simulink model "test_quadruped_staticwalk"  (R2018b)
settings: Solver=ode4  StartTime=0.0  StopTime=5  FixedStep=0.001  RelTol=1e-3  EnableMultiTasking=on
values from neighbouring files (symbols this model uses):
  Matlab_version = str2double(r_temp___(1))    [quadruped.m]
  Output_File = 'quadruped_demo1'    [quadruped.m]
  Output_file_n = r_temp___(2)    [quadruped.m]
  Plant_inputs_num = r_temp___(1)    [quadruped.m]
  Plant_outputs_num = r_temp___(1)    [quadruped.m]
  RecurDyn = 'C:\Program Files\FunctionBay, Inc\RecurDyn V9R1\Bin\'    [quadruped.m]
  RecurDyn_controltimestep = 1.e-003    (= 0.001)    [quadruped.m]
  RecurDyn_model = 'quadruped_demo1'    [quadruped.m]
  RecurDyn_model_n = r_temp___(2)    [quadruped.m]
settings Model: Creator=Administrator  LastModifiedBy=ahl19
settings OptimizationCC: LifeSpan=inf
settings DebuggingCC: SFUnexpectedBacktrackingDiag=warning  SFNoUnconditionalDefaultTransitionDiag=warning
settings SFSimCC: SimUseLocalCustomCode=off
settings RTWCC: RTWUseLocalCustomCode=off
settings CodeAppCC: StateflowObjectComments=on
settings GRTTargetCC: TargetLangStandard=C89/C90 (ANSI)  GeneratePreprocessorConditionals=Disable all
settings ConfigComp: CovMetricSettings=dw  CovHtmlReporting=on  CovSaveCumulativeToWorkspaceVar=on  CovSaveSingleToWorkspaceVar=on  CovExternalEMLEnable=off

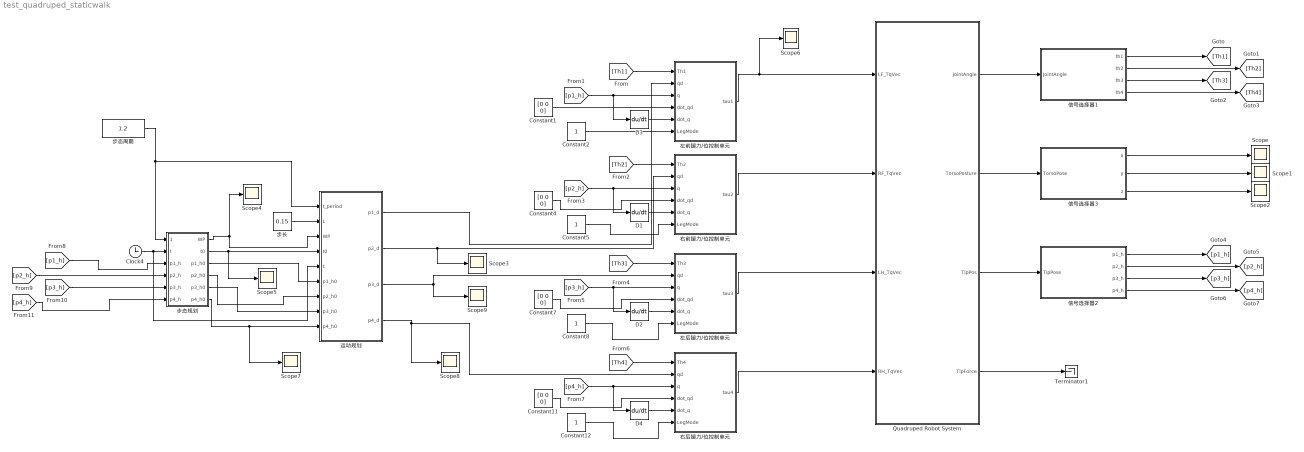
== system test_quadruped_staticwalk ==
  Clock4 : Clock
  Constant{1,4,7,11} (4 alike) : Constant  Value=[0 0 0]
  Constant{2,5,8,12} (4 alike) : Constant
  D{1..4} (4 alike) : Derivative  CoefficientInTFapproximation=0.01
  Quadruped Robot System : Subsystem
  Scope{,1..9} (10 alike) : Scope
  Terminator1 : Terminator
  信号选择器1 : MATLAB Function  TreatAsAtomicUnit=on
  信号选择器2 : MATLAB Function  TreatAsAtomicUnit=on
  信号选择器3 : MATLAB Function  TreatAsAtomicUnit=on
  右前腿力/位控制单元 : MATLAB Function  TreatAsAtomicUnit=on
  右后腿力/位控制单元 : MATLAB Function  TreatAsAtomicUnit=on
  左前腿力/位控制单元 : MATLAB Function  TreatAsAtomicUnit=on
  左后腿力/位控制单元 : MATLAB Function  TreatAsAtomicUnit=on
  步态周期 : Constant  Value=1.2
  步态规划 : MATLAB Function  TreatAsAtomicUnit=on
  步长 : Constant  Value=0.15
  运动规划 : MATLAB Function  TreatAsAtomicUnit=on
  wires:
  Quadruped Robot System/1(JointAngle) -> 信号选择器1/1(JointAngle)
  Quadruped Robot System/3(TipPos) -> 信号选择器2/1(TipPose)
  左前腿力/位控制单元/1(tau1) -> Scope6/1, Quadruped Robot System/1(LF_TqVec)
  右前腿力/位控制单元/1(tau2) -> Quadruped Robot System/2(RF_TqVec)
  左后腿力/位控制单元/1(tau3) -> Quadruped Robot System/3(LH_TqVec)
  右后腿力/位控制单元/1(tau4) -> Quadruped Robot System/4(RH_TqVec)
  信号选择器1/1(th1) -> [Th1]
  信号选择器1/2(th2) -> [Th2]
  信号选择器1/3(th3) -> [Th3]
  信号选择器1/4(th4) -> [Th4]
  [Th1] -> 左前腿力/位控制单元/1(Th1)
  信号选择器2/1(p1_h) -> [p1_h]
  信号选择器2/2(p2_h) -> [p2_h]
  信号选择器2/3(p3_h) -> [p3_h]
  信号选择器2/4(p4_h) -> [p4_h]
  [p1_h] -> D3/1, 左前腿力/位控制单元/3(q)
  Constant1/1 -> 左前腿力/位控制单元/4(dot_qd)
  D3/1 -> 左前腿力/位控制单元/5(dot_q)
  Constant2/1 -> 左前腿力/位控制单元/6(LegMode)
  [Th2] -> 右前腿力/位控制单元/1(Th2)
  [p2_h] -> 右前腿力/位控制单元/3(q), D1/1
  Constant4/1 -> 右前腿力/位控制单元/4(dot_qd)
  Constant5/1 -> 右前腿力/位控制单元/6(LegMode)
  [Th3] -> 左后腿力/位控制单元/1(Th3)
  [p3_h] -> 左后腿力/位控制单元/3(q), D2/1
  Constant7/1 -> 左后腿力/位控制单元/4(dot_qd)
  Constant8/1 -> 左后腿力/位控制单元/6(LegMode)
  D1/1 -> 右前腿力/位控制单元/5(dot_q)
  D2/1 -> 左后腿力/位控制单元/5(dot_q)
  [Th4] -> 右后腿力/位控制单元/1(Th4)
  [p4_h] -> 右后腿力/位控制单元/3(q), D4/1
  Constant11/1 -> 右后腿力/位控制单元/4(dot_qd)
  Constant12/1 -> 右后腿力/位控制单元/6(LegMode)
  D4/1 -> 右后腿力/位控制单元/5(dot_q)
  Quadruped Robot System/4(TipForce) -> Terminator1/1
  Quadruped Robot System/2(TorsoPosture) -> 信号选择器3/1(TorsoPose)
  信号选择器3/1(x) -> Scope/1
  信号选择器3/2(y) -> Scope1/1
  信号选择器3/3(z) -> Scope2/1
  Clock4/1 -> 步态规划/2(t), 运动规划/5(t)
  步态规划/1(WP) -> 运动规划/3(WP), Scope4/1
  步态规划/2(t0) -> Scope5/1, 运动规划/4(t0)
  步态周期/1 -> 运动规划/1(t_period), 步态规划/1(period)
  步长/1 -> 运动规划/2(L)
  [p1_h] -> 步态规划/3(p1_h)
  [p2_h] -> 步态规划/4(p2_h)
  [p3_h] -> 步态规划/5(p3_h)
  [p4_h] -> 步态规划/6(p4_h)
  步态规划/3(p1_h0) -> 运动规划/6(p1_h0)
  步态规划/4(p2_h0) -> 运动规划/7(p2_h0)
  步态规划/5(p3_h0) -> 运动规划/8(p3_h0)
  步态规划/6(p4_h0) -> Scope7/1, 运动规划/9(p4_h0)
  运动规划/1(p1_d) -> 左前腿力/位控制单元/2(qd)
  运动规划/2(p2_d) -> Scope3/1, 右前腿力/位控制单元/2(qd)
  运动规划/3(p3_d) -> Scope9/1, 左后腿力/位控制单元/2(qd)
  运动规划/4(p4_d) -> Scope8/1, 右后腿力/位控制单元/2(qd)

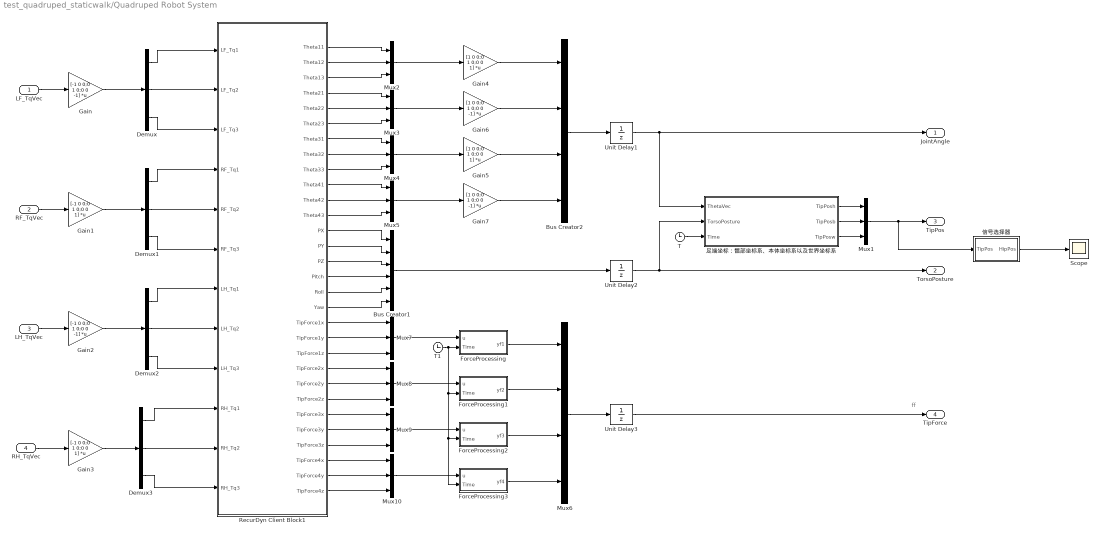
== system test_quadruped_staticwalk/Quadruped Robot System ==
  note: ff
  LF_TqVec : Inport
  RF_TqVec : Inport  Port=2
  LH_TqVec : Inport  Port=3
  RH_TqVec : Inport  Port=4
  Bus Creator1 : BusCreator  Inputs=6
  Bus Creator2 : BusCreator  Inputs=4
  Demux{,1..3} (4 alike) : Demux  Outputs=3
  ForceProcessing : MATLAB Function  TreatAsAtomicUnit=on
  ForceProcessing1 : MATLAB Function  TreatAsAtomicUnit=on
  ForceProcessing2 : MATLAB Function  TreatAsAtomicUnit=on
  ForceProcessing3 : MATLAB Function  TreatAsAtomicUnit=on
  Gain : Gain  Gain=[-1 0 0;0 1 0;0 0 -1]  Multiplication=Matrix(K*u) (u vector)
  Gain1 : Gain  Gain=[-1 0 0;0 1 0;0 0 1]  Multiplication=Matrix(K*u) (u vector)
  Gain2 : Gain  Gain=[-1 0 0;0 1 0;0 0 -1]  Multiplication=Matrix(K*u) (u vector)
  Gain3 : Gain  Gain=[-1 0 0;0 1 0;0 0 1]  Multiplication=Matrix(K*u) (u vector)
  Gain4 : Gain  Gain=[1 0 0;0 1 0;0 0 1]  Multiplication=Matrix(K*u) (u vector)
  Gain5 : Gain  Gain=[1 0 0;0 1 0;0 0 1]  Multiplication=Matrix(K*u) (u vector)
  Gain6 : Gain  Gain=[1 0 0;0 1 0;0 0 -1]  Multiplication=Matrix(K*u) (u vector)
  Gain7 : Gain  Gain=[1 0 0;0 1 0;0 0 -1]  Multiplication=Matrix(K*u) (u vector)
  Mux{1..5,7..10} (9 alike) : Mux  Inputs=3
  Mux6 : Mux
  RecurDyn Client Block1 : Subsystem
      mask Display: image(imread('RecurDyn_IF3x_Client.jpg'))
  Scope : Scope
  T : Clock
  T1 : Clock
  Unit Delay1 : UnitDelay  InitialCondition=[pi/2;pi/4;0;pi/2;pi/4;0;pi/2;pi/4;0;pi/2;pi/4;0]  SampleTime=0.001
  Unit Delay2 : UnitDelay  InitialCondition=[0;0.70;0;0;0;0]  SampleTime=0.001
  Unit Delay3 : UnitDelay  InitialCondition=[0;0;0;0;0;0;0;0;0;0;0;0]  SampleTime=0.001
  信号选择器 : MATLAB Function  TreatAsAtomicUnit=on
  足端坐标：髋部坐标系、本体坐标系以及世界坐标系 : MATLAB Function  TreatAsAtomicUnit=on
  JointAngle : Outport
  TorsoPosture : Outport  Port=2
  TipPos : Outport  Port=3
  TipForce : Outport  Port=4
  wires:
  Bus Creator2/1 -> Unit Delay1/1
  Mux1/1 -> 信号选择器/1(TipPos), TipPos/1
  足端坐标：髋部坐标系、本体坐标系以及世界坐标系/1(TipPosh) -> Mux1/1
  足端坐标：髋部坐标系、本体坐标系以及世界坐标系/2(TipPosb) -> Mux1/2
  足端坐标：髋部坐标系、本体坐标系以及世界坐标系/3(TipPosw) -> Mux1/3
  Unit Delay1/1 -> JointAngle/1, 足端坐标：髋部坐标系、本体坐标系以及世界坐标系/1(ThetaVec)
  Unit Delay3/1 -> TipForce/1
  Unit Delay2/1 -> TorsoPosture/1, 足端坐标：髋部坐标系、本体坐标系以及世界坐标系/2(TorsoPosture)
  Mux7/1 -> ForceProcessing/1(u)
  Mux8/1 -> ForceProcessing1/1(u)
  Mux9/1 -> ForceProcessing2/1(u)
  Mux10/1 -> ForceProcessing3/1(u)
  Gain/1 -> Demux/1
  LF_TqVec/1 -> Gain/1
  RF_TqVec/1 -> Gain1/1
  LH_TqVec/1 -> Gain2/1
  RH_TqVec/1 -> Gain3/1
  Mux2/1 -> Gain4/1
  Bus Creator1/1 -> Unit Delay2/1
  Demux/2 -> RecurDyn Client Block1/2(LF_Tq2)
  RecurDyn Client Block1/1("Theta11   ") -> Mux2/1
  RecurDyn Client Block1/2("Theta12   ") -> Mux2/2
  RecurDyn Client Block1/3("Theta13   ") -> Mux2/3
  RecurDyn Client Block1/4("Theta21   ") -> Mux3/1
  RecurDyn Client Block1/5("Theta22   ") -> Mux3/2
  RecurDyn Client Block1/6("Theta23   ") -> Mux3/3
  Mux3/1 -> Gain6/1
  RecurDyn Client Block1/7("Theta31   ") -> Mux4/1
  RecurDyn Client Block1/8("Theta32   ") -> Mux4/2
  RecurDyn Client Block1/9("Theta33   ") -> Mux4/3
  RecurDyn Client Block1/10("Theta41   ") -> Mux5/1
  RecurDyn Client Block1/11("Theta42   ") -> Mux5/2
  RecurDyn Client Block1/12("Theta43   ") -> Mux5/3
  Mux4/1 -> Gain5/1
  Mux5/1 -> Gain7/1
  Demux1/2 -> RecurDyn Client Block1/5(RF_Tq2)
  Demux1/1 -> RecurDyn Client Block1/4(RF_Tq1)
  Demux1/3 -> RecurDyn Client Block1/6(RF_Tq3)
  Demux/1 -> RecurDyn Client Block1/1(LF_Tq1)
  Demux/3 -> RecurDyn Client Block1/3(LF_Tq3)
  Gain1/1 -> Demux1/1
  Demux2/2 -> RecurDyn Client Block1/8(LH_Tq2)
  Demux2/1 -> RecurDyn Client Block1/7(LH_Tq1)
  Demux2/3 -> RecurDyn Client Block1/9(LH_Tq3)
  Gain2/1 -> Demux2/1
  Demux3/2 -> RecurDyn Client Block1/11(RH_Tq2)
  Demux3/1 -> RecurDyn Client Block1/10(RH_Tq1)
  Demux3/3 -> RecurDyn Client Block1/12(RH_Tq3)
  Gain3/1 -> Demux3/1
  RecurDyn Client Block1/19(TipForce1x) -> Mux7/1
  RecurDyn Client Block1/20(TipForce1y) -> Mux7/2
  RecurDyn Client Block1/21(TipForce1z) -> Mux7/3
  RecurDyn Client Block1/22(TipForce2x) -> Mux8/1
  RecurDyn Client Block1/23(TipForce2y) -> Mux8/2
  RecurDyn Client Block1/24(TipForce2z) -> Mux8/3
  RecurDyn Client Block1/25(TipForce3x) -> Mux9/1
  RecurDyn Client Block1/26(TipForce3y) -> Mux9/2
  RecurDyn Client Block1/27(TipForce3z) -> Mux9/3
  RecurDyn Client Block1/28(TipForce4x) -> Mux10/1
  RecurDyn Client Block1/29(TipForce4y) -> Mux10/2
  RecurDyn Client Block1/30(TipForce4z) -> Mux10/3
  RecurDyn Client Block1/13("PX        ") -> Bus Creator1/1
  RecurDyn Client Block1/14("PY        ") -> Bus Creator1/2
  RecurDyn Client Block1/15("PZ        ") -> Bus Creator1/3
  RecurDyn Client Block1/16("Pitch     ") -> Bus Creator1/4
  RecurDyn Client Block1/17("Roll      ") -> Bus Creator1/5
  RecurDyn Client Block1/18("Yaw       ") -> Bus Creator1/6
  Gain4/1 -> Bus Creator2/1
  Gain6/1 -> Bus Creator2/2
  Gain5/1 -> Bus Creator2/3
  Gain7/1 -> Bus Creator2/4
  Mux6/1 -> Unit Delay3/1
  T/1 -> 足端坐标：髋部坐标系、本体坐标系以及世界坐标系/3(Time)
  ForceProcessing/1(yf1) -> Mux6/1
  ForceProcessing1/1(yf2) -> Mux6/2
  ForceProcessing2/1(yf3) -> Mux6/3
  ForceProcessing3/1(yf4) -> Mux6/4
  T1/1 -> ForceProcessing/2(Time), ForceProcessing1/2(Time), ForceProcessing2/2(Time), ForceProcessing3/2(Time)
  信号选择器/1(HipPos) -> Scope/1

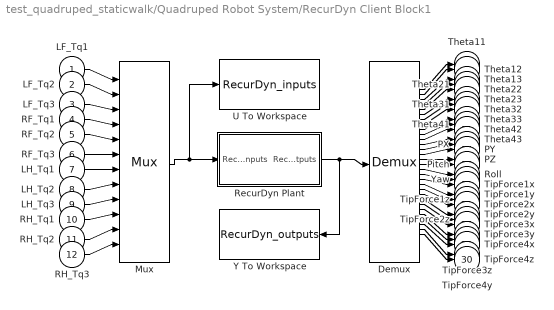
== system test_quadruped_staticwalk/Quadruped Robot System/RecurDyn Client Block1 ==
  LF_Tq1 : Inport
  LF_Tq2 : Inport  Port=2
  LF_Tq3 : Inport  Port=3
  RF_Tq1 : Inport  Port=4
  RF_Tq2 : Inport  Port=5
  RF_Tq3 : Inport  Port=6
  LH_Tq1 : Inport  Port=7
  LH_Tq2 : Inport  Port=8
  LH_Tq3 : Inport  Port=9
  RH_Tq1 : Inport  Port=10
  RH_Tq2 : Inport  Port=11
  RH_Tq3 : Inport  Port=12
  Demux : Demux  Outputs=30
  Mux : Mux  Inputs=12
  RecurDyn Plant : Subsystem  mask(Recurdyn/Plant){RecurDyn_model_name=RecurDyn_model, Output_File_Name_=Output_File, RecurDyn_=RecurDyn, Matlab_version_=Matlab_version, RecurDyn_controltimestep_=RecurDyn_controltimestep, RecurDyn_step_=100, Waitingtime=1000, RecurDyn_static_=off, RecurDyn_show_=on, RecurDyn_ani_=on, Create_Output_Folder_=off}
      mask prompts: Output_File_Name_ "Output File Name"; RecurDyn_ "RecurDyn_install_directory"; Matlab_version_ "Matlab version"; RecurDyn_controltimestep_ "Sampling period"; RecurDyn_step_ "RecurDyn_step"; Waitingtime "Waiting time"; RecurDyn_static_ "Static analysis"; RecurDyn_show_ "RecurDyn_show"; RecurDyn_ani_ "RecurDyn_animation"; Create_Output_Folder_ "Create Output Folder"
      mask help:
      | Simulate any Recurdyn Dynamics Model in Recurdyn/Solver
      | Plant inputs and Plant outputs are transfered every sampling time
      | Here, sampling time is determined by sampling period (Control time step)
      mask Display: disp( 'Dynamic Model' )
  U To Workspace : ToWorkspace  VariableName=RecurDyn_inputs
  Y To Workspace : ToWorkspace  VariableName=RecurDyn_outputs
  "Theta11   " : Outport
  "Theta12   " : Outport  Port=2
  "Theta13   " : Outport  Port=3
  "Theta21   " : Outport  Port=4
  "Theta22   " : Outport  Port=5
  "Theta23   " : Outport  Port=6
  "Theta31   " : Outport  Port=7
  "Theta32   " : Outport  Port=8
  "Theta33   " : Outport  Port=9
  "Theta41   " : Outport  Port=10
  "Theta42   " : Outport  Port=11
  "Theta43   " : Outport  Port=12
  "PX        " : Outport  Port=13
  "PY        " : Outport  Port=14
  "PZ        " : Outport  Port=15
  "Pitch     " : Outport  Port=16
  "Roll      " : Outport  Port=17
  "Yaw       " : Outport  Port=18
  TipForce1x : Outport  Port=19
  TipForce1y : Outport  Port=20
  TipForce1z : Outport  Port=21
  TipForce2x : Outport  Port=22
  TipForce2y : Outport  Port=23
  TipForce2z : Outport  Port=24
  TipForce3x : Outport  Port=25
  TipForce3y : Outport  Port=26
  TipForce3z : Outport  Port=27
  TipForce4x : Outport  Port=28
  TipForce4y : Outport  Port=29
  TipForce4z : Outport  Port=30
  wires:
  RecurDyn Plant/1(RecurDyn_outputs) -> Demux/1, Y To Workspace/1
  Mux/1 -> RecurDyn Plant/1(" RecurDyn_inputs"), U To Workspace/1
  Demux/1 -> "Theta11   "/1
  Demux/2 -> "Theta12   "/1
  Demux/3 -> "Theta13   "/1
  Demux/4 -> "Theta21   "/1
  Demux/5 -> "Theta22   "/1
  Demux/6 -> "Theta23   "/1
  Demux/7 -> "Theta31   "/1
  Demux/8 -> "Theta32   "/1
  Demux/9 -> "Theta33   "/1
  Demux/10 -> "Theta41   "/1
  Demux/11 -> "Theta42   "/1
  Demux/12 -> "Theta43   "/1
  Demux/13 -> "PX        "/1
  Demux/14 -> "PY        "/1
  Demux/15 -> "PZ        "/1
  Demux/16 -> "Pitch     "/1
  Demux/17 -> "Roll      "/1
  Demux/18 -> "Yaw       "/1
  Demux/19 -> TipForce1x/1
  Demux/20 -> TipForce1y/1
  Demux/21 -> TipForce1z/1
  Demux/22 -> TipForce2x/1
  Demux/23 -> TipForce2y/1
  Demux/24 -> TipForce2z/1
  Demux/25 -> TipForce3x/1
  Demux/26 -> TipForce3y/1
  Demux/27 -> TipForce3z/1
  Demux/28 -> TipForce4x/1
  Demux/29 -> TipForce4y/1
  Demux/30 -> TipForce4z/1
  LF_Tq1/1 -> Mux/1
  LF_Tq2/1 -> Mux/2
  LF_Tq3/1 -> Mux/3
  RF_Tq1/1 -> Mux/4
  RF_Tq2/1 -> Mux/5
  RF_Tq3/1 -> Mux/6
  LH_Tq1/1 -> Mux/7
  LH_Tq2/1 -> Mux/8
  LH_Tq3/1 -> Mux/9
  RH_Tq1/1 -> Mux/10
  RH_Tq2/1 -> Mux/11
  RH_Tq3/1 -> Mux/12

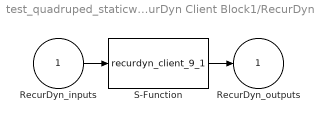
== system test_quadruped_staticwalk/Quadruped Robot System/RecurDyn Client Block1/RecurDyn Plant ==
  " RecurDyn_inputs" : Inport
  S-Function : S-Function  FunctionName=recurdyn_client_9_1  Parameters=RecurDyn_controltimestep_,RecurDyn_model_name,RecurDyn_,RecurDyn_static_,RecurDyn_step_,RecurDyn_show_,RecurDyn_ani_,Matlab_version_,RecurDyn_model_n,Plant_inputs_num,Plant_outputs_num,Waitingtime,Create_Output_Folder_,Output_File_Name_,Output_file_n  SFunctionDeploymentMode=off  EnableBusSupport=off
  RecurDyn_outputs : Outport  InitialOutput=0
  wires:
  S-Function/1 -> RecurDyn_outputs/1
  " RecurDyn_inputs"/1 -> S-Function/1

== matlab function test_quadruped_staticwalk/Quadruped Robot System/ForceProcessing1 ==
  data: u input; yf2 output; Time input
function yf2 = fp(u, Time)
% 处理足端力，y方向只提供大等于零的力
if Time<=0.001
    yf2 = zeros(3,1);
else
    yf2 = [1 0 0;0 (u(2)>=0) 0;0 0 1]*u;
end

end

== matlab function test_quadruped_staticwalk/Quadruped Robot System/ForceProcessing ==
  data: u input; yf1 output; Time input
function yf1 = fp(u, Time)
% 处理足端力，y方向只提供大等于零的力
if Time<=0.001
    yf1 = zeros(3,1);
else
    yf1 = [1 0 0;0 (u(2)>=0) 0;0 0 1]*u;
end

end

== matlab function test_quadruped_staticwalk/Quadruped Robot System/ForceProcessing2 ==
  data: u input; yf3 output; Time input
function yf3 = fp(u, Time)
% 处理足端力，y方向只提供大等于零的力
if Time<=0.001
    yf3 = zeros(3,1);
else
    yf3 = [1 0 0;0 (u(2)>=0) 0;0 0 1]*u;
end

end

== matlab function test_quadruped_staticwalk/Quadruped Robot System/ForceProcessing3 ==
  data: u input; yf4 output; Time input
function yf4 = fp(u, Time)
% 处理足端力，y方向只提供大等于零的力
if Time<=0.001
    yf4 = zeros(3,1);
else
    yf4 = [1 0 0;0 (u(2)>=0) 0;0 0 1]*u;
end

end

== matlab function test_quadruped_staticwalk/信号选择器2 ==
  data: TipPose input; p1_h output; p2_h output; p3_h output; p4_h output
function [p1_h,p2_h,p3_h,p4_h]  = SS(TipPose)

%% 
p1_h = TipPose(1:3);
p2_h = TipPose(4:6);
p3_h = TipPose(7:9);
p4_h = TipPose(10:12);


end

== matlab function test_quadruped_staticwalk/Quadruped Robot System/足端坐标：髋部坐标系、本体坐标系以及世界坐标系 ==
  data: ThetaVec input; TipPosh output; TipPosb output; TorsoPosture input; TipPosw output; Time input
function [TipPosh,TipPosb, TipPosw] = fk(ThetaVec, TorsoPosture, Time)

%% Notes
% 惯性系或世界坐标系：以机器人前进方向为【+X】，竖直向上为【+Y】，【+Z】由右手法则确定
% 本体固连坐标系：原点在质心处或几何中心，初始方向与惯性系一致
% 在髋部安装点处建立固连坐标系（方向与本体固连坐标系一致），计算足端位置（以下的顺序均为：左前、右前、左后、右后）

% BY ZPP
% 20171122

%% 设置仿真初值
if Time<=0.001
    ThetaVec = [pi/2;pi/4;0; pi/2;pi/4;0; pi/2;pi/4;0; pi/2;pi/4;0];
    TorsoPosture = [0; 0.70; 0;0;0;0];
end

%% 设置模型参数

% 重力加速度
g = 9.80665;

%本体尺寸的一半
L = 0.425; W = 0.19; H = -0.10 ;
% 本体质量
Mb = 50;

% 髋部安装点在本体固连坐标系中的坐标
A1 = [L -H -W]';
A2 = [L -H W]';
A3 = [-L -H -W]';
A4 = [-L -H W]';

Ab= [A1;A2;A3;A4];

% 单腿各连杆长度和质量
L1 = 0.35*sqrt(2);      % M1 = 1.0;
L2 = 0.35*sqrt(2);      % M2 = 1.5;
R3 = 0.06;                  % M3 = 0.5;

%% 输入关节角度
th11 = ThetaVec(1);
th12 = ThetaVec(2);
th13 = ThetaVec(3);

th21 = ThetaVec(4);
th22 = ThetaVec(5);
th23 = ThetaVec(6);

th31 = ThetaVec(7);
th32 = ThetaVec(8);
th33 = ThetaVec(9);

th41 = ThetaVec(10);
th42 = ThetaVec(11);
th43 = ThetaVec(12);

%% 正运动学1：计算髋部固连坐标系下足端的位置
x1 = L1*cos(th11 - th12) - L2*cos(th12);
y1 = - cos(th13)*(L2*sin(th12) + L1*sin(th11 - th12));
z1 = - sin(th13)*(L2*sin(th12) + L1*sin(th11 - th12));

x2 = L1*cos(th21 - th22) - L2*cos(th22);
y2 = - cos(th23)*(L2*sin(th22) + L1*sin(th21 - th22));
z2 = sin(th23)*(L2*sin(th22) + L1*sin(th21 - th22));

x3 = L1*cos(th31 - th32) - L2*cos(th32);
y3 = - cos(th33)*(L2*sin(th32) + L1*sin(th31 - th32));
z3 = - sin(th33)*(L2*sin(th32) + L1*sin(th31 - th32));

x4 = L1*cos(th41 - th42) - L2*cos(th42);
y4 = - cos(th43)*(L2*sin(th42) + L1*sin(th41 - th42));
z4 = sin(th43)*(L2*sin(th42) + L1*sin(th41 - th42));

TipPosh = [x1 y1 z1 x2 y2 z2 x3 y3 z3 x4 y4 z4]';

%% 正运动学2：计算本体固连坐标系下足端的位置
TipPosb = TipPosh + Ab;

%% 正运动学3：计算原点在本体质心处的惯性系下足端的位置
% 本体姿态角：Y-pitch / X-roll / Z-yaw
alpha = TorsoPosture(6); beta = TorsoPosture(4); gama = TorsoPosture(5);
RR = [cos(alpha)*cos(beta)  cos(alpha)*sin(beta)*sin(gama)-sin(alpha)*cos(gama)  cos(alpha)*sin(beta)*cos(gama)+sin(alpha)*sin(gama);...
         sin(alpha)*cos(beta)  sin(alpha)*sin(beta)*sin(gama)+cos(alpha)*cos(gama)  sin(alpha)*sin(beta)*cos(gama)-cos(alpha)*sin(gama);...
         -sin(beta)  cos(beta)*sin(gama)  cos(beta)*cos(gama)];
Rmat = blkdiag(RR,RR,RR,RR);
TipPosw = Rmat*TipPosb;

end

== matlab function test_quadruped_staticwalk/信号选择器3 ==
  data: TorsoPose input; x output; y output; z output
function [x,y,z]  = SS(TorsoPose)

%% 
x = TorsoPose(1);
y = TorsoPose(2);
z = TorsoPose(3);


end

== matlab function test_quadruped_staticwalk/右前腿力//位控制单元 ==
  data: Th2 input; qd input; q input; dot_qd input; dot_q input; LegMode input; tau2 output
%function [tau2,Fr]  = SLC(Th2,qd,q,dot_qd,dot_q,LegMode, Fwd,Fwf)
function tau2   = SLC(Th2,qd,q,dot_qd,dot_q,LegMode)

%% 关节角度、足端广义坐标以及雅克比矩阵的计算
th21=Th2(1);
th22=Th2(2);
th23=Th2(3);

% 单腿连杆参数
L1 = 0.35*sqrt(2);
L2 = 0.35*sqrt(2);
R3 = 0.06;

% Jacobian Matrix
J2 = [ -L1*sin(th21 - th22),                   L2*sin(th22) + L1*sin(th21 - th22),                      0;...
          -L1*cos(th21 - th22)*cos(th23), -cos(th23)*(L2*cos(th22) - L1*cos(th21 - th22)), sin(th23)*(L2*sin(th22) + L1*sin(th21 - th22));...
          L1*cos(th21 - th22)*sin(th23),   sin(th23)*(L2*cos(th22) - L1*cos(th21 - th22)),    cos(th23)*(L2*sin(th22) + L1*sin(th21 - th22))];

%% 初始化
 %Fr=zeros(3,1);
 %Fe = Fwf(4:6);    % 左前腿的足端接触力
 %Fd = Fwd(4:6);
 
tau2=zeros(3,1);

%% 单腿力/位控制模式
y = LegMode;
switch(y)
%%%%%%%%%%%%%%%%%%%%%%%%%%%%%
    

%%%%%%%%%%%%%%%%%%%%%%%%%%%%%
    case 1    % 单腿摆动
        kp = diag([8000 8000 8000]);
        kd = diag([500 500 500]);
        
        Fr=zeros(3,1);
        tau2=J2'*(kp*(qd-q)+kd*(dot_qd-dot_q)); 
        
%%%%%%%%%%%%%%%%%%%%%%%%%%%%%
    case 0    % 落后着地
        kp = diag([1000 1500 1000]);
        kd = diag([20 30 20]);
        
        % 在y方向上补偿0.01m
        qd1= qd+[0;-0.01;0];     
        Fr=zeros(3,1);
        tau2=J2'*(kp*(qd1-q)+kd*(dot_qd-dot_q));

%%%%%%%%%%%%%%%%%%%%%%%%%%%%%
     
end

%% 考虑实际情况：输出力矩限幅
Tmax = 500;

if tau2(1)>=Tmax
    tau2(1)=Tmax;
end
if tau2(1)<=-Tmax
    tau2(1)=-Tmax;
end
    
if tau2(2)>=Tmax
    tau2(2)=Tmax;
end
if tau2(2)<=-Tmax
    tau2(2)=-Tmax;
end
    
if tau2(3)>=Tmax
    tau2(3)=Tmax;
end
if tau2(3)<=-Tmax
    tau2(3)=-Tmax;
end

end

== matlab function test_quadruped_staticwalk/左后腿力//位控制单元 ==
  data: Th3 input; qd input; q input; dot_qd input; dot_q input; LegMode input; tau3 output
%function [tau3,Fr]  = SLC(Th3,qd,q,dot_qd,dot_q,LegMode, Fwd,Fwf)
function tau3   = SLC(Th3,qd,q,dot_qd,dot_q,LegMode)

%% 关节角度、足端广义坐标以及雅克比矩阵的计算
th31=Th3(1);
th32=Th3(2);
th33=Th3(3);

% 单腿连杆参数
L1 = 0.35*sqrt(2);
L2 = 0.35*sqrt(2);
R3 = 0.06;

% Jacobian Matrix
J3 = [ -L1*sin(th31 - th32),                   L2*sin(th32) + L1*sin(th31 - th32),                      0;...
          -L1*cos(th31 - th32)*cos(th33), -cos(th33)*(L2*cos(th32) - L1*cos(th31 - th32)), sin(th33)*(L2*sin(th32) + L1*sin(th31 - th32));...
          -L1*cos(th31 - th32)*sin(th33),  -sin(th33)*(L2*cos(th32) - L1*cos(th31 - th32)),  - cos(th33)*(L2*sin(th32) + L1*sin(th31 - th32))];

%% 初始化
 %Fr=zeros(3,1);
 %Fe = Fwf(7:9);    % 左前腿的足端接触力
 %Fd = Fwd(7:9);
 
tau3=zeros(3,1);

%% 单腿力/位控制模式
y = LegMode;
switch(y)
%%%%%%%%%%%%%%%%%%%%%%%%%%%%%
   

%%%%%%%%%%%%%%%%%%%%%%%%%%%%%
    case 1    % 单腿摆动
        kp = diag([8000 8000 8000]);
        kd = diag([500 500 500]);
        
        Fr=zeros(3,1);
        tau3=J3'*(kp*(qd-q)+kd*(dot_qd-dot_q)); 
        
%%%%%%%%%%%%%%%%%%%%%%%%%%%%%
    case 0    % 落后着地
        kp = diag([1000 1500 1000]);
        kd = diag([20 30 20]);
        
        % 在y方向上补偿0.01m
        qd1= qd+[0;-0.01;0];     
        Fr=zeros(3,1);
        tau3=J3'*(kp*(qd1-q)+kd*(dot_qd-dot_q));

%%%%%%%%%%%%%%%%%%%%%%%%%%%%%
     
end

%% 考虑实际情况：输出力矩限幅
Tmax = 500;

if tau3(1)>=Tmax
    tau3(1)=Tmax;
end
if tau3(1)<=-Tmax
    tau3(1)=-Tmax;
end
    
if tau3(2)>=Tmax
    tau3(2)=Tmax;
end
if tau3(2)<=-Tmax
    tau3(2)=-Tmax;
end
    
if tau3(3)>=Tmax
    tau3(3)=Tmax;
end
if tau3(3)<=-Tmax
    tau3(3)=-Tmax;
end

end

== matlab function test_quadruped_staticwalk/右后腿力//位控制单元 ==
  data: Th4 input; qd input; q input; dot_qd input; dot_q input; LegMode input; tau4 output
%function [tau4,Fr]  = SLC(Th4,qd,q,dot_qd,dot_q,LegMode, Fwd,Fwf)
function tau4   = SLC(Th4,qd,q,dot_qd,dot_q,LegMode)

%% 关节角度、足端广义坐标以及雅克比矩阵的计算
th41=Th4(1);
th42=Th4(2);
th43=Th4(3);

% 单腿连杆参数
L1 = 0.35*sqrt(2);
L2 = 0.35*sqrt(2);
R3 = 0.06;

% Jacobian Matrix
J4 = [ -L1*sin(th41 - th42),                   L2*sin(th42) + L1*sin(th41 - th42),                      0;...
          -L1*cos(th41 - th42)*cos(th43), -cos(th43)*(L2*cos(th42) - L1*cos(th41 - th42)), sin(th43)*(L2*sin(th42) + L1*sin(th41 - th42));...
          L1*cos(th41 - th42)*sin(th43),   sin(th43)*(L2*cos(th42) - L1*cos(th41 - th42)),    cos(th43)*(L2*sin(th42) + L1*sin(th41 - th42))];

%% 初始化
% Fr=zeros(3,1);
% Fe = Fwf(10:12);    % 左前腿的足端接触力
% Fd = Fwd(10:12);
 
tau4=zeros(3,1);

%% 单腿力/位控制模式
y = LegMode;
switch(y)
%%%%%%%%%%%%%%%%%%%%%%%%%%%%%
    

%%%%%%%%%%%%%%%%%%%%%%%%%%%%%
    case 1    % 单腿摆动
        kp = diag([8000 8000 8000]);
        kd = diag([500 500 500]);
        
        Fr=zeros(3,1);
        tau4=J4'*(kp*(qd-q)+kd*(dot_qd-dot_q)); 
        
%%%%%%%%%%%%%%%%%%%%%%%%%%%%%
    case 0    % 落后着地
        kp = diag([1000 1500 1000]);
        kd = diag([20 30 20]);
        
        % 在y方向上补偿0.01m
        qd1= qd+[0;-0.01;0];     
        Fr=zeros(3,1);
        tau4=J4'*(kp*(qd1-q)+kd*(dot_qd-dot_q));

%%%%%%%%%%%%%%%%%%%%%%%%%%%%%
     
end

%% 考虑实际情况：输出力矩限幅
Tmax = 500;

if tau4(1)>=Tmax
    tau4(1)=Tmax;
end
if tau4(1)<=-Tmax
    tau4(1)=-Tmax;
end
    
if tau4(2)>=Tmax
    tau4(2)=Tmax;
end
if tau4(2)<=-Tmax
    tau4(2)=-Tmax;
end
    
if tau4(3)>=Tmax
    tau4(3)=Tmax;
end
if tau4(3)<=-Tmax
    tau4(3)=-Tmax;
end

end

== matlab function test_quadruped_staticwalk/Quadruped Robot System/信号选择器 ==
  data: TipPos input; HipPos output
function HipPos  = SS(TipPos)

%% 
HipPos = TipPos(1:3);


end

== matlab function test_quadruped_staticwalk/左前腿力//位控制单元 ==
  data: Th1 input; qd input; q input; dot_qd input; dot_q input; LegMode input; tau1 output
%function [tau1,Fr, Fe]  = SLC(Th1,qd,q,dot_qd,dot_q,LegMode, Fwd,Fwf)
function tau1   = SLC(Th1,qd,q,dot_qd,dot_q,LegMode)

%% 关节角度、足端广义坐标以及雅克比矩阵的计算
th11=Th1(1);
th12=Th1(2);
th13=Th1(3);

% 单腿连杆参数
L1 = 0.35*sqrt(2);
L2 = 0.35*sqrt(2);
R3 = 0.06;

% Jacobian Matrix
J1 = [ -L1*sin(th11 - th12),                   L2*sin(th12) + L1*sin(th11 - th12),                      0;...
          -L1*cos(th11 - th12)*cos(th13), -cos(th13)*(L2*cos(th12) - L1*cos(th11 - th12)), sin(th13)*(L2*sin(th12) + L1*sin(th11 - th12));...
          -L1*cos(th11 - th12)*sin(th13),  -sin(th13)*(L2*cos(th12) - L1*cos(th11 - th12)),  - cos(th13)*(L2*sin(th12) + L1*sin(th11 - th12))];

%% 初始化
 %Fr=zeros(3,1);
 %Fe = Fwf(1:3);    % 左前腿的足端接触力
 %Fd = Fwd(1:3);
 
tau1=zeros(3,1);


%% 单腿力/位控制模式
y = LegMode;            %LegMode：0为落后着地模式；1为单腿摆动模式；2为单腿支撑模式；3为提前着地模式
switch(y)
%%%%%%%%%%%%%%%%%%%%%%%%%%%%%

%%%%%%%%%%%%%%%%%%%%%%%%%%%%%
    case 1    % 单腿摆动
        kp = diag([8000 8000 8000]);
        kd = diag([500 500 500]);
        
        Fr=zeros(3,1);
        tau1=J1'*(kp*(qd-q)+kd*(dot_qd-dot_q)); 
        
%%%%%%%%%%%%%%%%%%%%%%%%%%%%%
    case 0    % 落后着地
        kp = diag([1000 1500 1000]);
        kd = diag([20 30 20]);
        
        % 在y方向上补偿0.01m
        qd1= qd+[0;-0.01;0];     
        Fr=zeros(3,1);
        tau1=J1'*(kp*(qd1-q)+kd*(dot_qd-dot_q));

%%%%%%%%%%%%%%%%%%%%%%%%%%%%%
     
end

%% 考虑实际情况：输出力矩限幅
Tmax = 500;

if tau1(1)>=Tmax
    tau1(1)=Tmax;
end
if tau1(1)<=-Tmax
    tau1(1)=-Tmax;
end
    
if tau1(2)>=Tmax
    tau1(2)=Tmax;
end
if tau1(2)<=-Tmax
    tau1(2)=-Tmax;
end
    
if tau1(3)>=Tmax
    tau1(3)=Tmax;
end
if tau1(3)<=-Tmax
    tau1(3)=-Tmax;
end

end

== matlab function test_quadruped_staticwalk/信号选择器1 ==
  data: JointAngle input; th1 output; th2 output; th3 output; th4 output
function [th1,th2,th3,th4]  = SS(JointAngle)

%% 
th1 = JointAngle(1:3);
th2 = JointAngle(4:6);
th3 = JointAngle(7:9);
th4 = JointAngle(10:12);


end

== matlab function test_quadruped_staticwalk/步态规划 ==
  data: period input; t input; WP output; t0 output; p1_h input; p2_h input; p3_h input; p4_h input; p1_h0 output; p2_h0 output; p3_h0 output; p4_h0 output
function [WP,t0,p1_h0,p2_h0,p3_h0,p4_h0] = walkpattern(period,t,p1_h,p2_h,p3_h,p4_h)
%#codegen

persistent tmp_WP;
persistent tmp_t0;
if isempty(tmp_WP)
    tmp_WP = 0;
end
if isempty(tmp_t0)
    tmp_t0 = 0;
end

persistent tmp_p1_h0;
persistent tmp_p2_h0;
persistent tmp_p3_h0;
persistent tmp_p4_h0;
if isempty(tmp_p1_h0)
    tmp_p1_h0 = [0 -0.7 0];
end
if isempty(tmp_p2_h0)
    tmp_p2_h0 = [0 -0.7 0];
end
if isempty(tmp_p3_h0)
    tmp_p3_h0 = [0 -0.7 0];
end
if isempty(tmp_p4_h0)
    tmp_p4_h0 = [0 -0.7 0];
end

t_tmp = period/6;                   %整个步态周期分为6步

if t<period
    tmp_WP = 10;
    tmp_t0 = 0;
else
    t_period = mod(t,period);

    if t_period<t_tmp
        if t<(period+t_tmp)
            tmp_t0 = period;
            tmp_WP = 0;             %首次质心位移
            
            tmp_p1_h0 = [0 -0.7 0];
            tmp_p2_h0 = [0 -0.7 0];
            tmp_p3_h0 = [0 -0.7 0];
            tmp_p4_h0 = [0 -0.7 0];
        else
            if tmp_WP ~= 6
                tmp_t0 = t;
                tmp_WP = 6;             %31运动后四足支撑
                
                tmp_p1_h0 = [p1_h(1) -0.7 p1_h(3)];
                tmp_p2_h0 = [p2_h(1) -0.7 p2_h(3)];
                tmp_p3_h0 = [p3_h(1) -0.7 p3_h(3)];
                tmp_p4_h0 = [p4_h(1) -0.7 p4_h(3)];
            end
        end
    else if t_period<(2*t_tmp)
            if tmp_WP ~= 4
                tmp_t0 = t;
                tmp_WP = 4;             %4腿摆动
                
                tmp_p1_h0 = [p1_h(1) -0.7 p1_h(3)];
                tmp_p2_h0 = [p2_h(1) -0.7 p2_h(3)];
                tmp_p3_h0 = [p3_h(1) -0.7 p3_h(3)];
                tmp_p4_h0 = [p4_h(1) -0.7 p4_h(3)];
            end
        else if t_period<(3*t_tmp)
                if tmp_WP ~= 2
                    tmp_t0 = t;
                    tmp_WP = 2;             %2腿摆动
                    
                    tmp_p1_h0 = [p1_h(1) -0.7 p1_h(3)];
                    tmp_p2_h0 = [p2_h(1) -0.7 p2_h(3)];
                    tmp_p3_h0 = [p3_h(1) -0.7 p3_h(3)];
                    tmp_p4_h0 = [p4_h(1) -0.7 p4_h(3)];
                end
            else if t_period<(4*t_tmp)
                    if tmp_WP ~= 5
                        tmp_t0 = t;
                        tmp_WP = 5;             %42运动后四足支撑
                        
                        tmp_p1_h0 = [p1_h(1) -0.7 p1_h(3)];
                        tmp_p2_h0 = [p2_h(1) -0.7 p2_h(3)];
                        tmp_p3_h0 = [p3_h(1) -0.7 p3_h(3)];
                        tmp_p4_h0 = [p4_h(1) -0.7 p4_h(3)];
                    end
                else if t_period<(5*t_tmp)
                        if tmp_WP ~= 3
                            tmp_t0 = t;
                            tmp_WP = 3;             %3腿摆动
                            
                            tmp_p1_h0 = [p1_h(1) -0.7 p1_h(3)];
                            tmp_p2_h0 = [p2_h(1) -0.7 p2_h(3)];
                            tmp_p3_h0 = [p3_h(1) -0.7 p3_h(3)];
                            tmp_p4_h0 = [p4_h(1) -0.7 p4_h(3)];
                        end
                    else if t_period<(6*t_tmp)
                            if tmp_WP ~= 1
                                tmp_t0 = t;
                                tmp_WP = 1;             %1腿摆动
                                
                                tmp_p1_h0 = [p1_h(1) -0.7 p1_h(3)];
                                tmp_p2_h0 = [p2_h(1) -0.7 p2_h(3)];
                                tmp_p3_h0 = [p3_h(1) -0.7 p3_h(3)];
                                tmp_p4_h0 = [p4_h(1) -0.7 p4_h(3)];
                            end
                        else
                            WP = 0;
                            t0 = period;
                        end
                    end
                end
            end
        end
    end
end

WP = tmp_WP;
t0 = tmp_t0;

p1_h0 = tmp_p1_h0;
p2_h0 = tmp_p2_h0;
p3_h0 = tmp_p3_h0;
p4_h0 = tmp_p4_h0;

== matlab function test_quadruped_staticwalk/运动规划 ==
  data: t_period input; L input; WP input; p1_d output; t0 input; t input; p2_d output; p3_d output; p4_d output; p1_h0 input; p2_h0 input; p3_h0 input; p4_h0 input
function [p1_d,p2_d,p3_d,p4_d] = motionplan(t_period,L,WP,t0,t,p1_h0,p2_h0,p3_h0,p4_h0)
%#codegen

p1_d = zeros(3,1);
p2_d = zeros(3,1);
p3_d = zeros(3,1);
p4_d = zeros(3,1);

t_tmp = t_period/6;                   %整个步态周期分为6步

switch(WP)
    case 0                          %起始阶段，质心移动[0.5*L 0 -L]。
        x_d0 = 0;
        y_d0 = -0.7;
        z_d0 = 0;
        
        x_end = -0.5*L;            %腿部动作与质心动作相反。
        y_end = -0.7;
        z_end = 0.05;
        
        x_delta = x_end - x_d0;
        y_delta = y_end - y_d0;
        z_delta = z_end - z_d0;

        x1_d = x_d0 + x_delta*(1-cos(pi*(t-t0)/t_tmp))*0.5;
        y1_d = y_d0 + y_delta*sin(pi*(t-t0)/t_tmp);
        z1_d = z_d0 + z_delta*(1-cos(pi*(t-t0)/t_tmp))*0.5;
        
        x2_d = x_d0 + x_delta*(1-cos(pi*(t-t0)/t_tmp))*0.5;
        y2_d = y_d0 + y_delta*sin(pi*(t-t0)/t_tmp);
        z2_d = z_d0 + z_delta*(1-cos(pi*(t-t0)/t_tmp))*0.5;
        
        x3_d = x_d0 + x_delta*(1-cos(pi*(t-t0)/t_tmp))*0.5;
        y3_d = y_d0 + y_delta*sin(pi*(t-t0)/t_tmp);
        z3_d = z_d0 + z_delta*(1-cos(pi*(t-t0)/t_tmp))*0.5;
        
        x4_d = x_d0 + x_delta*(1-cos(pi*(t-t0)/t_tmp))*0.5;
        y4_d = y_d0 + y_delta*sin(pi*(t-t0)/t_tmp);
        z4_d = z_d0 + z_delta*(1-cos(pi*(t-t0)/t_tmp))*0.5;
        
    case 4                      %4腿摆动
        x1_d = p1_h0(1);
        y1_d = p1_h0(2);
        z1_d = p1_h0(3);
        
        x2_d = p2_h0(1);
        y2_d = p2_h0(2);
        z2_d = p2_h0(3);
        
        x3_d = p3_h0(1);
        y3_d = p3_h0(2);
        z3_d = p3_h0(3);
        
        x4_d0 = p4_h0(1);
        y4_d0 = p4_h0(2);
        z4_d0 = p4_h0(3);
        
        x4_end = L;            %腿部动作。
        y4_end = -0.7;
        z4_end = 0.05;
        
        x4_delta = x4_end - x4_d0;
        %y4_delta = y4_end - y4_d0;
        y4_delta = 0.1;
        z4_delta = z4_end - z4_d0;
        
        x4_d = x4_d0 + x4_delta*(1-cos(pi*(t-t0)/t_tmp))*0.5;
        y4_d = y4_d0 + y4_delta*sin(pi*(t-t0)/t_tmp);
        z4_d = z4_d0 + z4_delta*(1-cos(pi*(t-t0)/t_tmp))*0.5;
        
    case 2                      %2腿摆动
        x1_d = p1_h0(1);
        y1_d = p1_h0(2);
        z1_d = p1_h0(3);
        
        x3_d = p3_h0(1);
        y3_d = p3_h0(2);
        z3_d = p3_h0(3);
        
        x4_d = p4_h0(1);
        y4_d = p4_h0(2);
        z4_d = p4_h0(3);
        
        x2_d0 = p2_h0(1);
        y2_d0 = p2_h0(2);
        z2_d0 = p2_h0(3);
        
        x2_end = L;            %腿部动作与质心动作相反。
        y2_end = -0.7;
        z2_end = 0.05;
        
        x2_delta = x2_end - x2_d0;
        %y2_delta = y2_end - y2_d0;
        y2_delta = 0.1;
        z2_delta = z2_end - z2_d0;
        
        x2_d = x2_d0 + x2_delta*(1-cos(pi*(t-t0)/t_tmp))*0.5;
        y2_d = y2_d0 + y2_delta*sin(pi*(t-t0)/t_tmp);
        z2_d = z2_d0 + z2_delta*(1-cos(pi*(t-t0)/t_tmp))*0.5;

    case 5                              %42腿摆动后，质心移动[0.2 0 0.2]
        x1_d0 = p1_h0(1);
        y1_d0 = p1_h0(2);
        z1_d0 = p1_h0(3);
        
        x2_d0 = p2_h0(1);
        y2_d0 = p2_h0(2);
        z2_d0 = p2_h0(3);
        
        x3_d0 = p3_h0(1);
        y3_d0 = p3_h0(2);
        z3_d0 = p3_h0(3);
        
        x4_d0 = p4_h0(1);
        y4_d0 = p4_h0(2);
        z4_d0 = p4_h0(3);
        
        x1_end = -1.5*L;            %腿部动作与质心动作相反。
        y1_end = -0.7;
        z1_end = -0.05;
        
        x2_end = -L;            %腿部动作与质心动作相反。
        y2_end = -0.7;
        z2_end = -0.05;
        
        x3_end = -1.5*L;            %腿部动作与质心动作相反。
        y3_end = -0.7;
        z3_end = -0.05;
        
        x4_end = -L;            %腿部动作与质心动作相反。
        y4_end = -0.7;
        z4_end = -0.05;
        
        x1_delta = x1_end - x1_d0;
        y1_delta = y1_end - y1_d0;
        z1_delta = z1_end - z1_d0;
        
        x2_delta = x2_end - x2_d0;
        y2_delta = y2_end - y2_d0;
        z2_delta = z2_end - z2_d0;
        
        x3_delta = x3_end - x3_d0;
        y3_delta = y3_end - y3_d0;
        z3_delta = z3_end - z3_d0;
        
        x4_delta = x4_end - x4_d0;
        y4_delta = y4_end - y4_d0;
        z4_delta = z4_end - z4_d0;
        
        x1_d = x1_d0 + x1_delta*(1-cos(pi*(t-t0)/t_tmp))*0.5;
        y1_d = y1_d0 + y1_delta*sin(pi*(t-t0)/t_tmp);
        z1_d = z1_d0 + z1_delta*(1-cos(pi*(t-t0)/t_tmp))*0.5;
        
        x2_d = x2_d0 + x2_delta*(1-cos(pi*(t-t0)/t_tmp))*0.5;
        y2_d = y2_d0 + y2_delta*sin(pi*(t-t0)/t_tmp);
        z2_d = z2_d0 + z2_delta*(1-cos(pi*(t-t0)/t_tmp))*0.5;
        
        x3_d = x3_d0 + x3_delta*(1-cos(pi*(t-t0)/t_tmp))*0.5;
        y3_d = y3_d0 + y3_delta*sin(pi*(t-t0)/t_tmp);
        z3_d = z3_d0 + z3_delta*(1-cos(pi*(t-t0)/t_tmp))*0.5;
        
        x4_d = x4_d0 + x4_delta*(1-cos(pi*(t-t0)/t_tmp))*0.5;
        y4_d = y4_d0 + y4_delta*sin(pi*(t-t0)/t_tmp);
        z4_d = z4_d0 + z4_delta*(1-cos(pi*(t-t0)/t_tmp))*0.5;
        
    case 3                      %3腿摆动
        x1_d = p1_h0(1);
        y1_d = p1_h0(2);
        z1_d = p1_h0(3);
        
        x2_d = p2_h0(1);
        y2_d = p2_h0(2);
        z2_d = p2_h0(3);
        
        x4_d = p4_h0(1);
        y4_d = p4_h0(2);
        z4_d = p4_h0(3);
        
        x3_d0 = p3_h0(1);
        y3_d0 = p3_h0(2);
        z3_d0 = p3_h0(3);
        
        x3_end = L;            %腿部动作与质心动作相反。
        y3_end = -0.7;
        z3_end = -0.05;
        
        x3_delta = x3_end - x3_d0;
        %y3_delta = y3_end - y3_d0;
        y3_delta = 0.1;
        z3_delta = z3_end - z3_d0;
        
        x3_d = x3_d0 + x3_delta*(1-cos(pi*(t-t0)/t_tmp))*0.5;
        y3_d = y3_d0 + y3_delta*sin(pi*(t-t0)/t_tmp);
        z3_d = z3_d0 + z3_delta*(1-cos(pi*(t-t0)/t_tmp))*0.5;
        
    case 1                      %1腿摆动
        x2_d = p2_h0(1);
        y2_d = p2_h0(2);
        z2_d = p2_h0(3);
        
        x3_d = p3_h0(1);
        y3_d = p3_h0(2);
        z3_d = p3_h0(3);
        
        x4_d = p4_h0(1);
        y4_d = p4_h0(2);
        z4_d = p4_h0(3);
        
        x1_d0 = p1_h0(1);
        y1_d0 = p1_h0(2);
        z1_d0 = p1_h0(3);
        
        x1_end = L;            %腿部动作与质心动作相反。
        y1_end = -0.7;
        z1_end = -0.05;
        
        x1_delta = x1_end - x1_d0;
        y1_delta = y1_end - y1_d0;
        z1_delta = z1_end - z1_d0;
        
        x1_d = x1_d0 + x1_delta*(1-cos(pi*(t-t0)/t_tmp))*0.5;
        y1_d = y1_d0 + y1_delta*sin(pi*(t-t0)/t_tmp);
        z1_d = z1_d0 + z1_delta*(1-cos(pi*(t-t0)/t_tmp))*0.5;
        
    case 6                              %31腿摆动后，质心移动[0.1 0 -0.1]
        x1_d0 = p1_h0(1);
        y1_d0 = p1_h0(2);
        z1_d0 = p1_h0(3);
        
        x2_d0 = p2_h0(1);
        y2_d0 = p2_h0(2);
        z2_d0 = p2_h0(3);
        
        x3_d0 = p3_h0(1);
        y3_d0 = p3_h0(2);
        z3_d0 = p3_h0(3);
        
        x4_d0 = p4_h0(1);
        y4_d0 = p4_h0(2);
        z4_d0 = p4_h0(3);
        
        x1_end = -L;            %腿部动作与质心动作相反。
        y1_end = -0.7;
        z1_end = 0.05;
        
        x2_end = -1.5*L;            %腿部动作与质心动作相反。
        y2_end = -0.7;
        z2_end = 0.05;
        
        x3_end = -L;            %腿部动作与质心动作相反。
        y3_end = -0.7;
        z3_end = 0.05;
        
        x4_end = -1.5*L;            %腿部动作与质心动作相反。
        y4_end = -0.7;
        z4_end = 0.05;
        
        x1_delta = x1_end - x1_d0;
        y1_delta = y1_end - y1_d0;
        z1_delta = z1_end - z1_d0;
        
        x2_delta = x2_end - x2_d0;
        y2_delta = y2_end - y2_d0;
        z2_delta = z2_end - z2_d0;
        
        x3_delta = x3_end - x3_d0;
        y3_delta = y3_end - y3_d0;
        z3_delta = z3_end - z3_d0;
        
        x4_delta = x4_end - x4_d0;
        y4_delta = y4_end - y4_d0;
        z4_delta = z4_end - z4_d0;
        
        x1_d = x1_d0 + x1_delta*(1-cos(pi*(t-t0)/t_tmp))*0.5;
        y1_d = y1_d0 + y1_delta*sin(pi*(t-t0)/t_tmp);
        z1_d = z1_d0 + z1_delta*(1-cos(pi*(t-t0)/t_tmp))*0.5;
        
        x2_d = x2_d0 + x2_delta*(1-cos(pi*(t-t0)/t_tmp))*0.5;
        y2_d = y2_d0 + y2_delta*sin(pi*(t-t0)/t_tmp);
        z2_d = z2_d0 + z2_delta*(1-cos(pi*(t-t0)/t_tmp))*0.5;
        
        x3_d = x3_d0 + x3_delta*(1-cos(pi*(t-t0)/t_tmp))*0.5;
        y3_d = y3_d0 + y3_delta*sin(pi*(t-t0)/t_tmp);
        z3_d = z3_d0 + z3_delta*(1-cos(pi*(t-t0)/t_tmp))*0.5;
        
        x4_d = x4_d0 + x4_delta*(1-cos(pi*(t-t0)/t_tmp))*0.5;
        y4_d = y4_d0 + y4_delta*sin(pi*(t-t0)/t_tmp);
        z4_d = z4_d0 + z4_delta*(1-cos(pi*(t-t0)/t_tmp))*0.5;
        
    otherwise
        x1_d = p1_h0(1);
        y1_d = p1_h0(2);
        z1_d = p1_h0(3);
        
        x2_d = p2_h0(1);
        y2_d = p2_h0(2);
        z2_d = p2_h0(3);
        
        x3_d = p3_h0(1);
        y3_d = p3_h0(2);
        z3_d = p3_h0(3);
        
        x4_d = p4_h0(1);
        y4_d = p4_h0(2);
        z4_d = p4_h0(3);
end


p1_d(1) = x1_d;
p1_d(2) = y1_d;
p1_d(3) = z1_d;

p2_d(1) = x2_d;
p2_d(2) = y2_d;
p2_d(3) = z2_d;

p3_d(1) = x3_d;
p3_d(2) = y3_d;
p3_d(3) = z3_d;

p4_d(1) = x4_d;
p4_d(2) = y4_d;
p4_d(3) = z4_d;
